simulink model "sldemo_lct_inherit_dims"  (Simulink 7.6)
settings: Solver=FixedStepDiscrete  StartTime=0.0  StopTime=10.0  FixedStep=1  RelTol=1e-3
values from neighbouring files (symbols this model uses):
  p1 = block.FixedPointNumericType(dt1)    [msfcn_complex_multip_fi.m]    (also in msfcn_frame_filt.m = block.DialogPrm(1).Data; msfcn_frame_gen.m = block.DialogPrm(1).Data)
  p2 = block.FixedPointNumericType(dt2)    [msfcn_complex_multip_fi.m]    (also in msfcn_frame_filt.m = block.DialogPrm(2).Data; msfcn_frame_gen.m = sprintf(')
  p3 = sprintf('    [msfcn_frame_gen.m]
Description:
  | Inherited Signal Dimensions
settings Model: Creator=The MathWorks Inc.  ExtModeAutoUpdateStatusClock=off
settings DataIOCC: SaveOutput=off  SaveTime=off  SignalLoggingName=logsOut
settings OptimizationCC: InlineParams=on  InlineInvariantSignals=on  ZeroExternalMemoryAtStartup=off  ZeroInternalMemoryAtStartup=off  NoFixptDivByZeroProtection=on  EfficientFloat2IntCast=on  OptimizeModelRefInitCode=on  LifeSpan=1
settings DebuggingCC: SaveWithParameterizedLinksMsg=none  SolverPrmCheckMsg=none  MultiTaskDSMMsg=warning  SignalLabelMismatchMsg=warning  RootOutportRequireBusObject=none
settings HardwareCC: ProdIntDivRoundTo=Floor  TargetEndianess=LittleEndian  TargetHWDeviceType=MATLAB Host
settings RTWCC: SystemTargetFile=ert.tlc  GenCodeOnly=on  TemplateMakefile=ert_default_tmf  Description=RTW Embedded Coder (no auto configuration)  GenerateReport=on  ProcessScript=ert_make_rtw_hook  IncludeHyperlinkInReport=on  LaunchReport=on  IncludeERTFirstTime=on
settings CodeAppCC: IgnoreCustomStorageClasses=off
settings ERTTargetCC: TargetFcnLib=ansi_tfl_tmw.mat  MultiwordLength=2048  GenerateSampleERTMain=on  IncludeMdlTerminateFcn=off  SuppressErrorStatus=on  InlinedParameterPlacement=NonHierarchical  ERTSrcFileBannerTemplate=example_banner.tlc  ERTHdrFileBannerTemplate=example_banner.tlc  ERTCustomFileTemplate=example_file_process.tlc  ConvertIfToSwitch=off

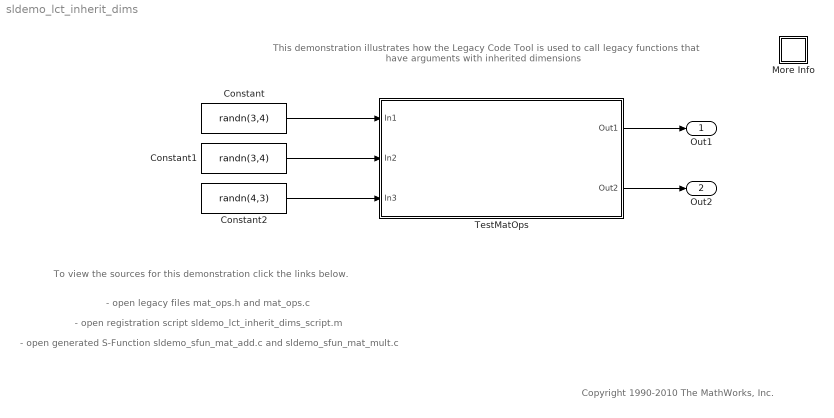
== system sldemo_lct_inherit_dims ==
  note: Copyright 1990-2010 The MathWorks, Inc.
  note: This demonstration illustrates how the Legacy Code Tool is used to
      | call legacy functions that have arguments with inherited dimensions
  note: - open legacy files mat_ops.h and mat_ops.c
  note: To view the sources for this demonstration
      | click the links below.
  note: - open registration script sldemo_lct_inherit_dims_script.m
  note: - open generated S-Function sldemo_sfun_mat_add.c and sldemo_sfun_mat_mult.c
  Constant : Constant  Value=randn(3,4)  OutDataTypeStr=double
  Constant1 : Constant  Value=randn(3,4)  OutDataTypeStr=double
  Constant2 : Constant  Value=randn(4,3)  OutDataTypeStr=double
  More Info : Subsystem
      settings: OpenFcn=showdemo('sldemo_lct_inherit_dims_script')
      mask Display: disp('?')
  TestMatOps : Subsystem
  Out1 : Outport
  Out2 : Outport  Port=2
  wires:
  TestMatOps/1(Out1) -> Out1/1
  Constant/1 -> TestMatOps/1(In1)
  Constant1/1 -> TestMatOps/2(In2)
  Constant2/1 -> TestMatOps/3(In3)
  TestMatOps/2(Out2) -> Out2/1

== system sldemo_lct_inherit_dims/More Info ==

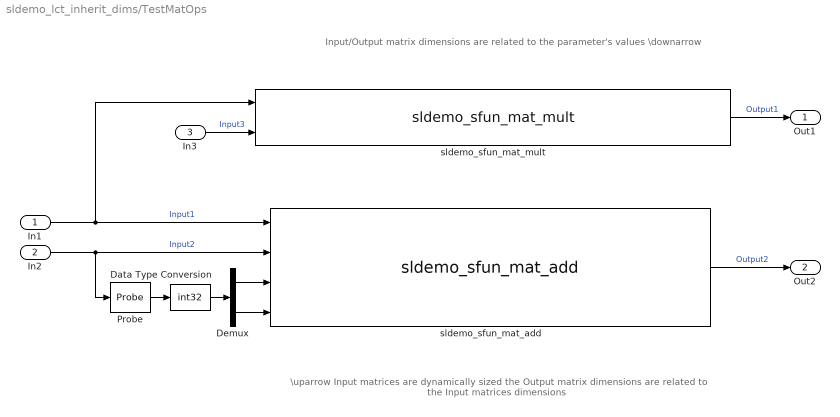
== system sldemo_lct_inherit_dims/TestMatOps ==
  note: Input/Output matrix dimensions are related to the parameter's values
      | \downarrow
  note: \uparrow
      | Input matrices are dynamically sized
      | the Output matrix dimensions are related to the Input matrices dimensions
  In1 : Inport
  In2 : Inport  Port=2
  In3 : Inport  Port=3
  Data Type Conversion : DataTypeConversion  OutDataTypeStr=int32
  Demux : Demux  Outputs=2
  Probe : Probe  ProbeWidth=off  ProbeSampleTime=off  ProbeComplexSignal=off  ProbeSignalDimensions=on
  sldemo_sfun_mat_add : S-Function  FunctionName=sldemo_sfun_mat_add  EnableBusSupport=off  mask(Legacy Function){SFunctionSpec=void mat_add(double u1[][], double u2[][], int32 u3, int32 u4, double y1[size(u1,1)][size(u1,2)]), ShowSpec=on}
      mask prompts: ShowSpec "Display function specification"
      mask help:
      | This block allows you to call the legacy functions specified by the following Legacy Code Tool definition:
      | def.SFunctionName = 'sldemo_sfun_mat_add';
      | def.OutputFcnSpec = 'void mat_add(double u1[][], double u2[][], int32 u3, int32 u4, double y1[size(u1,1)][size(u1,2)])';
      | def.HeaderFiles = {'mat_ops.h'};
      | def.SourceFiles = {'mat_ops.c'};
      | def.IncPaths = {'sldemo_lct_src'};
      | def.SrcPaths = {'sldemo_lct_src'};
      mask Help: <p>This block was generated automatically by the Legacy Code Tool. For detailed help on this tool, call<a href="matlab:legacy_code('help')"> legacy_code('help')</a>.</p>
      mask CallbackString:
      | |if strcmp(get_param(gcbh, 'ShowSpec'), 'on')
      |   set_param(gcbh, 'MaskDisplay', sprintf('fprintf(''%s'');', get_param(gcbh, 'SFunctionSpec')));
      | else
      |   set_param(gcbh, 'MaskDisplay', sprintf('fprintf(''%s'');', get_param(gcbh, 'FunctionName')));
      | end
      mask Display: fprintf('void mat_add(double u1[][], double u2[][], int32 u3, int32 u4, double y1[size(u1,1)][size(u1,2)])');
  sldemo_sfun_mat_mult : S-Function  FunctionName=sldemo_sfun_mat_mult  Parameters=SParameter1, SParameter2, SParameter3  EnableBusSupport=off  mask(Legacy Function){SFunctionSpec=void mat_mult(double u1[p1][p2], double u2[p2][p3], int32 p1, int32 p2, int32 p3, double y1[p1][p3]), SParameter1=int32(3), SParameter2=int32(4), SParameter3=int32(3), ShowSpec=on}
      mask prompts: SParameter1 "P1:"; SParameter2 "P2:"; SParameter3 "P3:"; ShowSpec "Display function specification"
      mask help:
      | This block allows you to call the legacy functions specified by the following Legacy Code Tool definition:
      | def.SFunctionName = 'sldemo_sfun_mat_mult';
      | def.OutputFcnSpec = 'void mat_mult(double u1[p1][p2], double u2[p2][p3], int32 p1, int32 p2, int32 p3, double y1[p1][p3])';
      | def.HeaderFiles = {'mat_ops.h'};
      | def.SourceFiles = {'mat_ops.c'};
      | def.IncPaths = {'sldemo_lct_src'};
      | def.SrcPaths = {'sldemo_lct_src'};
      mask Help: <p>This block was generated automatically by the Legacy Code Tool. For detailed help on this tool, call<a href="matlab:legacy_code('help')"> legacy_code('help')</a>.</p>
      mask CallbackString:
      | ||||if strcmp(get_param(gcbh, 'ShowSpec'), 'on')
      |   set_param(gcbh, 'MaskDisplay', sprintf('fprintf(''%s'');', get_param(gcbh, 'SFunctionSpec')));
      | else
      |   set_param(gcbh, 'MaskDisplay', sprintf('fprintf(''%s'');', get_param(gcbh, 'FunctionName')));
      | end
      mask Display: fprintf('void mat_mult(double u1[p1][p2], double u2[p2][p3], int32 p1, int32 p2, int32 p3, double y1[p1][p3])');
  Out1 : Outport
  Out2 : Outport  Port=2
  wires:
  In2/1 -> Probe/1, sldemo_sfun_mat_add/2  "Input2"
  sldemo_sfun_mat_add/1 -> Out2/1  "Output2"
  In1/1 -> sldemo_sfun_mat_mult/1, sldemo_sfun_mat_add/1  "Input1"
  Data Type Conversion/1 -> Demux/1
  Probe/1 -> Data Type Conversion/1
  Demux/2 -> sldemo_sfun_mat_add/4
  Demux/1 -> sldemo_sfun_mat_add/3
  In3/1 -> sldemo_sfun_mat_mult/2  "Input3"
  sldemo_sfun_mat_mult/1 -> Out1/1  "Output1"
